simulink model "ABS_simulation"  (R2022b)
settings: Solver=VariableStepAuto  StartTime=0.0  StopTime=10  RelTol=1e-3
libraries: simulink x1
settings Model: Creator=rahulchakravarthula  LastModifiedBy=rahulchakravarthula

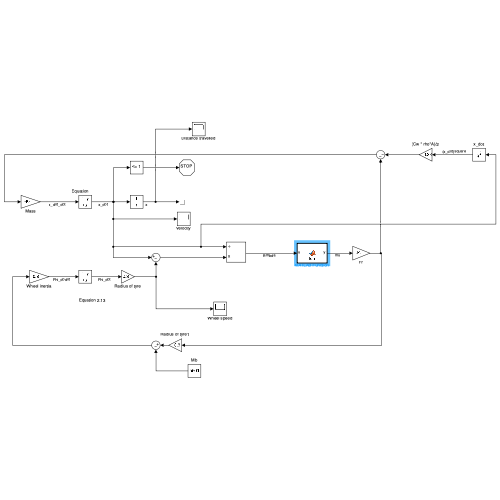
[thumbnail: Simulink's stored preview of the top-level diagram]
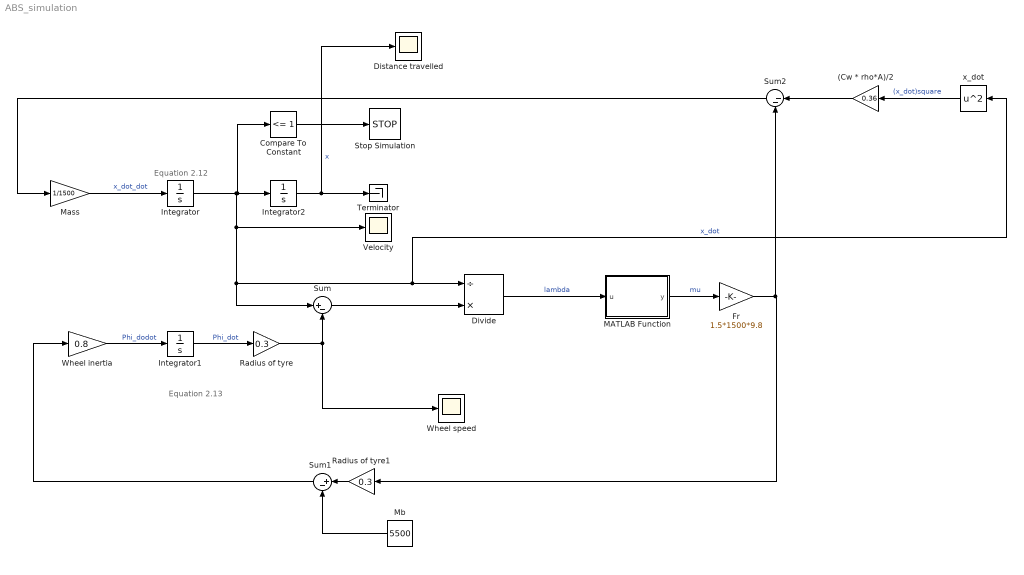
== system ABS_simulation ==
  note: Equation 2.12
  note: Equation 2.13
  (Cw * rho*A)/2 : Gain  Gain=0.36
  Compare To Constant : simulink/Logic and Bit Operations/Compare To Constant  relop=<=  const=1  OutDataTypeStr=boolean
  Distance travelled : Scope
  Divide : Product  Inputs=/*
  Fr : Gain  Gain=1.5*1500*9.8
  Integrator : Integrator  InitialCondition=100/3.6  LimitOutput=on  LowerSaturationLimit=0
  Integrator1 : Integrator  InitialCondition=(100/3.6)/0.3  LimitOutput=on  LowerSaturationLimit=0
  Integrator2 : Integrator  LowerSaturationLimit=0
  MATLAB Function : MATLAB Function  TreatAsAtomicUnit=on
  Mass : Gain  Gain=1/1500
  Mb : Constant  Value=5500
  Radius of tyre : Gain  Gain=0.3
  Radius of tyre1 : Gain  Gain=0.3
  Stop Simulation : Stop
  Sum : Sum  Inputs=|+-
  Sum1 : Sum  Inputs=|+-
  Sum2 : Sum  Inputs=|--
  Terminator : Terminator
  Velocity : Scope
  Wheel inertia : Gain  Gain=0.8
  Wheel speed : Scope
  x_dot : Math  Operator=square
  wires:
  Mass/1 -> Integrator/1  "x_dot_dot"
  Integrator/1 -> Compare To Constant/1, Integrator2/1, Sum/1, x_dot/1, Divide/1, Velocity/1  "x_dot"
  Integrator2/1 -> Distance travelled/1, Terminator/1  "x"
  Integrator1/1 -> Radius of tyre/1  "Phi_dot"
  Wheel inertia/1 -> Integrator1/1  "Phi_dodot"
  Radius of tyre/1 -> Wheel speed/1, Sum/2
  Sum/1 -> Divide/2
  Divide/1 -> MATLAB Function/1(u)  "lambda"
  MATLAB Function/1(y) -> Fr/1  "mu"
  Fr/1 -> Radius of tyre1/1, Sum2/2
  Radius of tyre1/1 -> Sum1/1
  Mb/1 -> Sum1/2
  Sum1/1 -> Wheel inertia/1
  x_dot/1 -> (Cw * rho*A)/2/1  "(x_dot)square"
  (Cw * rho*A)/2/1 -> Sum2/1
  Sum2/1 -> Mass/1
  Compare To Constant/1 -> Stop Simulation/1

== matlab function ABS_simulation/MATLAB Function ==
  data: u input; y output
function y = fcn(u)

c1 = 0.86;
c2 = 33.82;
c3 = 0.36;

y = c1*(1-exp(-c2*u)) - c3*u;
